simulink model "block_diagram_for_three_phase_csi"  (R2014a)
settings: Solver=ode23t  StartTime=0  StopTime=1  MaxStep=1e-6  RelTol=1e-3
values from neighbouring files (symbols this model uses):
  p11 = rem(m,360)    [code_for_single_phase_csi.m]    (also in code_for_single_phase_vsi.m; code_for_three_phase_csi.m; code_for_three_phase_vsi.m; code_for_vsi.m)
  p22 = rem(n,360)    [code_for_single_phase_csi.m]    (also in code_for_single_phase_vsi.m; code_for_three_phase_csi.m; code_for_three_phase_vsi.m; code_for_vsi.m)
  p33 = rem(o,360)    [code_for_single_phase_csi.m]    (also in code_for_single_phase_vsi.m; code_for_three_phase_csi.m; code_for_three_phase_vsi.m; code_for_vsi.m)
  p44 = rem(p,360)    [code_for_single_phase_csi.m]    (also in code_for_single_phase_vsi.m; code_for_three_phase_csi.m; code_for_three_phase_vsi.m; code_for_vsi.m)
  p55 = rem(q,360)    [code_for_single_phase_csi.m]    (also in code_for_single_phase_vsi.m; code_for_three_phase_csi.m; code_for_three_phase_vsi.m; code_for_vsi.m)
  p66 = rem(r,360)    [code_for_single_phase_csi.m]    (also in code_for_single_phase_vsi.m; code_for_three_phase_csi.m; code_for_three_phase_vsi.m; code_for_vsi.m)
  p77 = rem(s,360)    [code_for_single_phase_csi.m]    (also in code_for_single_phase_vsi.m; code_for_three_phase_csi.m; code_for_three_phase_vsi.m; code_for_vsi.m)
libraries: powerlib x14, powerlib_meascontrol x2
settings Model: Creator=singa  LastModifiedBy=singa

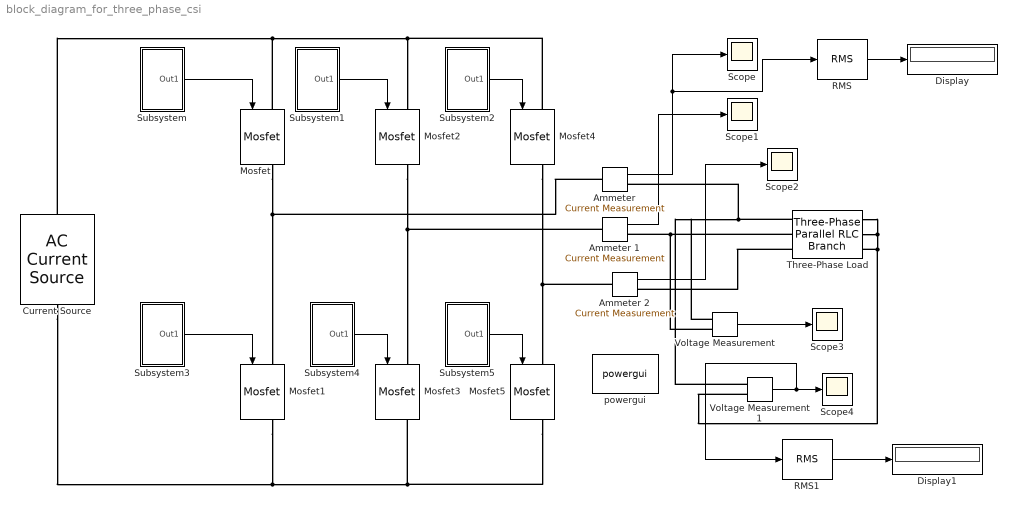
== system block_diagram_for_three_phase_csi ==
  Ammeter : powerlib/Measurements/Current Measurement  PhasorSimulation=off  OutputType=Complex  PSBequivalent=0
  Ammeter 1 : powerlib/Measurements/Current Measurement  PhasorSimulation=off  OutputType=Complex  PSBequivalent=0
  Ammeter 2 : powerlib/Measurements/Current Measurement  PhasorSimulation=off  OutputType=Complex  PSBequivalent=0
  Current Source : powerlib/Electrical Sources/AC Current Source  Amplitude=200  Phase=90  Frequency=0  SampleTime=0  Measurements=None
  Display : Display
  Display1 : Display
  Mosfet{,1..5} (6 alike) : powerlib/Power Electronics/Mosfet  Ron=0.1  Lon=0  Rd=0.01  Vfd=0  IC=0  Rs=1e5  Cs=inf  Measurements=on
  RMS : powerlib_meascontrol/Measurements/RMS  TrueRMS=on  Freq=50  RMSInit=120  Ts=0
  RMS1 : powerlib_meascontrol/Measurements/RMS  TrueRMS=on  Freq=50  RMSInit=120  Ts=0
  Scope{,1..4} (5 alike) : Scope
      Scope settings: YMin=-8  YMax=8  SampleInput=on  SampleTime=1e-6
      Scope1 settings: YMin=-8  YMax=8  SampleInput=on  SampleTime=1e-6
      Scope2 settings: YMin=-8  YMax=8  SaveName=ScopeData2  SampleInput=on  SampleTime=1e-6
      Scope3 settings: YMin=-8  YMax=8  SaveName=ScopeData3  SampleInput=on  SampleTime=1e-6
      Scope4 settings: YMin=-8  YMax=8  SaveName=ScopeData4  SampleInput=on  SampleTime=1e-6
  Subsystem : Subsystem
  Subsystem1 : Subsystem
  Subsystem2 : Subsystem
  Subsystem3 : Subsystem
  Subsystem4 : Subsystem
  Subsystem5 : Subsystem
  Three-Phase Load : powerlib/Elements/Three-Phase Parallel RLC Branch  LConnTagsString=A|B|C  RConnTagsString=A|B|C  BranchType=RC  Resistance=1  Inductance=1e-3  Capacitance=0.1  Measurements=None
  Voltage Measurement : powerlib/Measurements/Voltage Measurement  PhasorSimulation=off  OutputType=Complex  PSBequivalent=0
  Voltage Measurement1 : powerlib/Measurements/Voltage Measurement  PhasorSimulation=off  OutputType=Complex  PSBequivalent=0
  powergui : powerlib/powergui  Priority=1  SimulationMode=Continuous  SolverType=Tustin  SampleTime=50e-6  frequency=60  SPID=off  DisableSnubberDevices=off  DisableRonSwitches=off  DisableVfSwitches=off  SwTol=0  Interpol=off  DisplayEquations=off  Ts=0  methode=off  frequencyindice=0  Pbase=100e6  ErrMax=1e-4  Iterations=50  UnitsV=kV  UnitsW=MW  FunctionMessages=off  echomessages=off  HookPort=off  EnableUseOfTLC=off  x0status=blocks  RestoreLinks=warning  ResistiveCurrentMeasurement=off  Frange=[0:2:500]  Ylog=off  Xlog=on  ShowGrid=off  save=off  variable=ZData  structure=ScopeData  ZoomFFT=off  StartTime=0.8  cycles=2  DisplayStyle=4  fundamental=50  FreqAxis=on  MaxFrequency=2500  frequencyindicesteady=1  RmsSteady=1  display=off
  wires:
  Ammeter/1 -> Scope/1, RMS/1
  Ammeter 1/1 -> Scope1/1
  Ammeter 2/1 -> Scope2/1
  Subsystem/1(Out1) -> Mosfet/1
  Subsystem1/1(Out1) -> Mosfet2/1
  Subsystem2/1(Out1) -> Mosfet4/1
  Subsystem3/1(Out1) -> Mosfet1/1
  Subsystem4/1(Out1) -> Mosfet3/1
  Subsystem5/1(Out1) -> Mosfet5/1
  Voltage Measurement/1 -> Scope3/1
  Voltage Measurement1/1 -> RMS1/1, Scope4/1
  RMS1/1 -> Display1/1
  RMS/1 -> Display/1
  connections:
  Mosfet/RConn1 -- Mosfet1/LConn1 -- Ammeter/LConn1
  Mosfet2/RConn1 -- Mosfet3/LConn1 -- Ammeter 1/LConn1
  Mosfet4/RConn1 -- Ammeter 2/LConn1 -- Mosfet5/LConn1
  Mosfet/LConn1 -- Mosfet4/LConn1 -- Mosfet2/LConn1 -- Current Source/RConn1
  Mosfet1/RConn1 -- Mosfet5/RConn1 -- Mosfet3/RConn1 -- Current Source/LConn1
  Three-Phase Load/LConn1 -- Voltage Measurement1/LConn1 -- Voltage Measurement/LConn1 -- Ammeter/RConn1
  Three-Phase Load/LConn2 -- Voltage Measurement/LConn2 -- Ammeter 1/RConn1
  Three-Phase Load/LConn3 -- Ammeter 2/RConn1
  Three-Phase Load/RConn1 -- Three-Phase Load/RConn2 -- Voltage Measurement1/LConn2 -- Three-Phase Load/RConn3

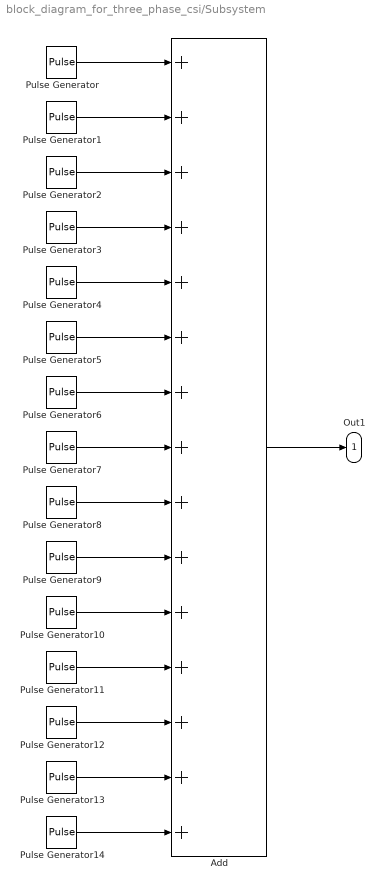
== system block_diagram_for_three_phase_csi/Subsystem ==
  Add : Sum  Inputs=+++++++++++++++
  Pulse Generator : DiscretePulseGenerator  PulseType=Time based  Period=0.02  PulseWidth=(p22-p11)/360*100  PhaseDelay=p11/360*0.02
  Pulse Generator1 : DiscretePulseGenerator  PulseType=Time based  Period=0.02  PulseWidth=(p55-p44)/360*100  PhaseDelay=p44/360*0.02
  Pulse Generator10 : DiscretePulseGenerator  PulseType=Time based  Period=0.02  PulseWidth=(p22-p11)/360*100  PhaseDelay=(180-p22)/360*0.02
  Pulse Generator11 : DiscretePulseGenerator  PulseType=Time based  Period=0.02  PulseWidth=(p33-p22)/360*100  PhaseDelay=(240+p22)/360*0.02
  Pulse Generator12 : DiscretePulseGenerator  PulseType=Time based  Period=0.02  PulseWidth=(p66-p55)/360*100  PhaseDelay=(240+p55)/360*0.02
  Pulse Generator13 : DiscretePulseGenerator  PulseType=Time based  Period=0.02  PulseWidth=(p66-p55)/360*100  PhaseDelay=(300-p66)/360*0.02
  Pulse Generator14 : DiscretePulseGenerator  PulseType=Time based  Period=0.02  PulseWidth=(p33-p22)/360*100  PhaseDelay=(300-p33)/360*0.02
  Pulse Generator2 : DiscretePulseGenerator  PulseType=Time based  Period=0.02  PulseWidth=(30-p77)/360*100  PhaseDelay=p77/360*0.02
  Pulse Generator3 : DiscretePulseGenerator  PulseType=Time based  Period=0.02  PulseWidth=(p77-p66)/360*100  PhaseDelay=(60-p77)/360*0.02
  Pulse Generator4 : DiscretePulseGenerator  PulseType=Time based  Period=0.02  PulseWidth=(p44-p33)/360*100  PhaseDelay=(60-p44)/360*0.02
  Pulse Generator5 : DiscretePulseGenerator  PulseType=Time based  Period=0.02  PulseWidth=(30+p11)/180*100  PhaseDelay=(60-p11)/360*0.02
  Pulse Generator6 : DiscretePulseGenerator  PulseType=Time based  Period=0.02  PulseWidth=(p44-p33)/360*100  PhaseDelay=(120+p33)/360*0.02
  Pulse Generator7 : DiscretePulseGenerator  PulseType=Time based  Period=0.02  PulseWidth=(p77-p66)/360*100  PhaseDelay=(120+p66)/360*0.02
  Pulse Generator8 : DiscretePulseGenerator  PulseType=Time based  Period=0.02  PulseWidth=(30-p77)/360*100  PhaseDelay=150/360*0.02
  Pulse Generator9 : DiscretePulseGenerator  PulseType=Time based  Period=0.02  PulseWidth=(p55-p44)/360*100  PhaseDelay=(180-p55)/360*0.02
  Out1 : Outport
  wires:
  Add/1 -> Out1/1
  Pulse Generator2/1 -> Add/3
  Pulse Generator/1 -> Add/1
  Pulse Generator1/1 -> Add/2
  Pulse Generator3/1 -> Add/4
  Pulse Generator9/1 -> Add/10
  Pulse Generator13/1 -> Add/14
  Pulse Generator14/1 -> Add/15
  Pulse Generator12/1 -> Add/13
  Pulse Generator6/1 -> Add/7
  Pulse Generator7/1 -> Add/8
  Pulse Generator4/1 -> Add/5
  Pulse Generator8/1 -> Add/9
  Pulse Generator11/1 -> Add/12
  Pulse Generator5/1 -> Add/6
  Pulse Generator10/1 -> Add/11

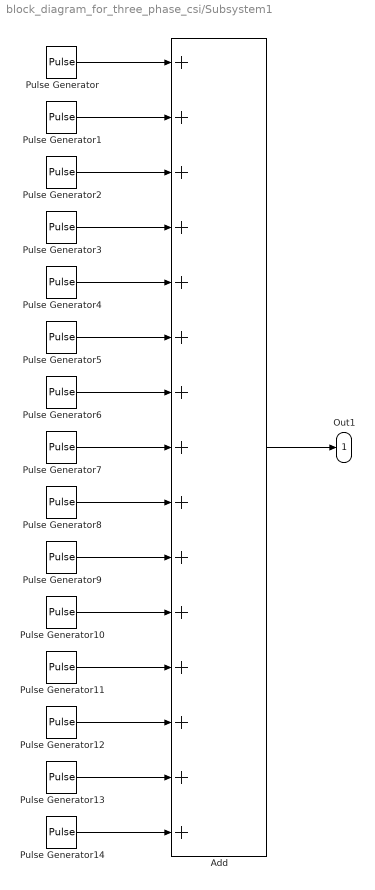
== system block_diagram_for_three_phase_csi/Subsystem1 ==
  Add : Sum  Inputs=+++++++++++++++
  Pulse Generator : DiscretePulseGenerator  PulseType=Time based  Period=0.02  PulseWidth=(p22-p11)/360*100  PhaseDelay=p11/360*0.02+0.02/3
  Pulse Generator1 : DiscretePulseGenerator  PulseType=Time based  Period=0.02  PulseWidth=(p55-p44)/360*100  PhaseDelay=p44/360*0.02+0.02/3
  Pulse Generator10 : DiscretePulseGenerator  PulseType=Time based  Period=0.02  PulseWidth=(p22-p11)/360*100  PhaseDelay=(180-p22)/360*0.02+0.02/3
  Pulse Generator11 : DiscretePulseGenerator  PulseType=Time based  Period=0.02  PulseWidth=(p33-p22)/360*100  PhaseDelay=(240+p22)/360*0.02+0.02/3
  Pulse Generator12 : DiscretePulseGenerator  PulseType=Time based  Period=0.02  PulseWidth=(p66-p55)/360*100  PhaseDelay=(240+p55)/360*0.02+0.02/3
  Pulse Generator13 : DiscretePulseGenerator  PulseType=Time based  Period=0.02  PulseWidth=(p66-p55)/360*100  PhaseDelay=(300-p66)/360*0.02+0.02/3
  Pulse Generator14 : DiscretePulseGenerator  PulseType=Time based  Period=0.02  PulseWidth=(p33-p22)/360*100  PhaseDelay=(300-p33)/360*0.02+0.02/3
  Pulse Generator2 : DiscretePulseGenerator  PulseType=Time based  Period=0.02  PulseWidth=(30-p77)/360*100  PhaseDelay=p77/360*0.02+0.02/3
  Pulse Generator3 : DiscretePulseGenerator  PulseType=Time based  Period=0.02  PulseWidth=(p77-p66)/360*100  PhaseDelay=(60-p77)/360*0.02+0.02/3
  Pulse Generator4 : DiscretePulseGenerator  PulseType=Time based  Period=0.02  PulseWidth=(p44-p33)/360*100  PhaseDelay=(60-p44)/360*0.02+0.02/3
  Pulse Generator5 : DiscretePulseGenerator  PulseType=Time based  Period=0.02  PulseWidth=(30+p11)/180*100  PhaseDelay=(60-p11)/360*0.02+0.02/3
  Pulse Generator6 : DiscretePulseGenerator  PulseType=Time based  Period=0.02  PulseWidth=(p44-p33)/360*100  PhaseDelay=(120+p33)/360*0.02+0.02/3
  Pulse Generator7 : DiscretePulseGenerator  PulseType=Time based  Period=0.02  PulseWidth=(p77-p66)/360*100  PhaseDelay=(120+p66)/360*0.02+0.02/3
  Pulse Generator8 : DiscretePulseGenerator  PulseType=Time based  Period=0.02  PulseWidth=(30-p77)/360*100  PhaseDelay=150/360*0.02+0.02/3
  Pulse Generator9 : DiscretePulseGenerator  PulseType=Time based  Period=0.02  PulseWidth=(p55-p44)/360*100  PhaseDelay=(180-p55)/360*0.02+0.02/3
  Out1 : Outport
  wires:
  Pulse Generator2/1 -> Add/3
  Pulse Generator/1 -> Add/1
  Pulse Generator1/1 -> Add/2
  Pulse Generator3/1 -> Add/4
  Pulse Generator9/1 -> Add/10
  Pulse Generator13/1 -> Add/14
  Pulse Generator14/1 -> Add/15
  Pulse Generator12/1 -> Add/13
  Pulse Generator6/1 -> Add/7
  Pulse Generator7/1 -> Add/8
  Pulse Generator4/1 -> Add/5
  Pulse Generator8/1 -> Add/9
  Pulse Generator11/1 -> Add/12
  Pulse Generator5/1 -> Add/6
  Pulse Generator10/1 -> Add/11
  Add/1 -> Out1/1

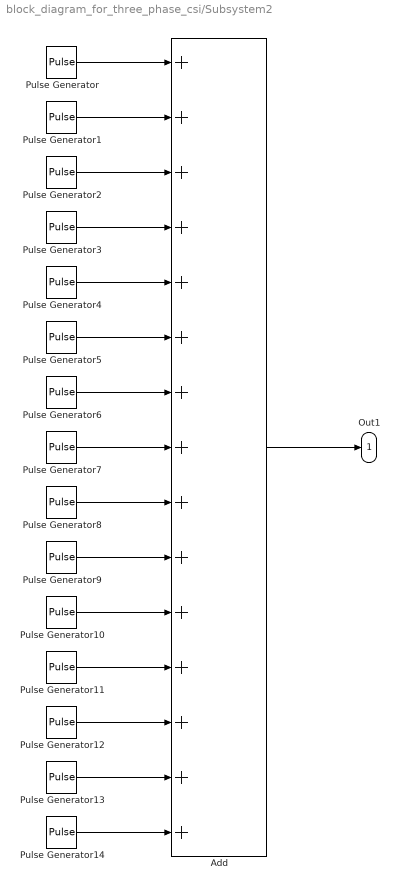
== system block_diagram_for_three_phase_csi/Subsystem2 ==
  Add : Sum  Inputs=+++++++++++++++
  Pulse Generator : DiscretePulseGenerator  PulseType=Time based  Period=0.02  PulseWidth=(p22-p11)/360*100  PhaseDelay=p11/360*0.02+0.04/3
  Pulse Generator1 : DiscretePulseGenerator  PulseType=Time based  Period=0.02  PulseWidth=(p55-p44)/360*100  PhaseDelay=p44/360*0.02+0.04/3
  Pulse Generator10 : DiscretePulseGenerator  PulseType=Time based  Period=0.02  PulseWidth=(p22-p11)/360*100  PhaseDelay=(180-p22)/360*0.02+0.04/3
  Pulse Generator11 : DiscretePulseGenerator  PulseType=Time based  Period=0.02  PulseWidth=(p33-p22)/360*100  PhaseDelay=(240+p22)/360*0.02+0.04/3
  Pulse Generator12 : DiscretePulseGenerator  PulseType=Time based  Period=0.02  PulseWidth=(p66-p55)/360*100  PhaseDelay=(240+p55)/360*0.02+0.04/3
  Pulse Generator13 : DiscretePulseGenerator  PulseType=Time based  Period=0.02  PulseWidth=(p66-p55)/360*100  PhaseDelay=(300-p66)/360*0.02+0.04/3
  Pulse Generator14 : DiscretePulseGenerator  PulseType=Time based  Period=0.02  PulseWidth=(p33-p22)/360*100  PhaseDelay=(300-p33)/360*0.02+0.04/3
  Pulse Generator2 : DiscretePulseGenerator  PulseType=Time based  Period=0.02  PulseWidth=(30-p77)/360*100  PhaseDelay=p77/360*0.02+0.04/3
  Pulse Generator3 : DiscretePulseGenerator  PulseType=Time based  Period=0.02  PulseWidth=(p77-p66)/360*100  PhaseDelay=(60-p77)/360*0.02+0.04/3
  Pulse Generator4 : DiscretePulseGenerator  PulseType=Time based  Period=0.02  PulseWidth=(p44-p33)/360*100  PhaseDelay=(60-p44)/360*0.02+0.04/3
  Pulse Generator5 : DiscretePulseGenerator  PulseType=Time based  Period=0.02  PulseWidth=(30+p11)/180*100  PhaseDelay=(60-p11)/360*0.02+0.04/3
  Pulse Generator6 : DiscretePulseGenerator  PulseType=Time based  Period=0.02  PulseWidth=(p44-p33)/360*100  PhaseDelay=(120+p33)/360*0.02+0.04/3
  Pulse Generator7 : DiscretePulseGenerator  PulseType=Time based  Period=0.02  PulseWidth=(p77-p66)/360*100  PhaseDelay=(120+p66)/360*0.02+0.04/3
  Pulse Generator8 : DiscretePulseGenerator  PulseType=Time based  Period=0.02  PulseWidth=(30-p77)/360*100  PhaseDelay=150/360*0.02+0.04/3
  Pulse Generator9 : DiscretePulseGenerator  PulseType=Time based  Period=0.02  PulseWidth=(p55-p44)/360*100  PhaseDelay=(180-p55)/360*0.02+0.04/3
  Out1 : Outport
  wires:
  Pulse Generator2/1 -> Add/3
  Pulse Generator/1 -> Add/1
  Pulse Generator1/1 -> Add/2
  Pulse Generator3/1 -> Add/4
  Pulse Generator9/1 -> Add/10
  Pulse Generator13/1 -> Add/14
  Pulse Generator14/1 -> Add/15
  Pulse Generator12/1 -> Add/13
  Pulse Generator6/1 -> Add/7
  Pulse Generator7/1 -> Add/8
  Pulse Generator4/1 -> Add/5
  Pulse Generator8/1 -> Add/9
  Pulse Generator11/1 -> Add/12
  Pulse Generator5/1 -> Add/6
  Pulse Generator10/1 -> Add/11
  Add/1 -> Out1/1

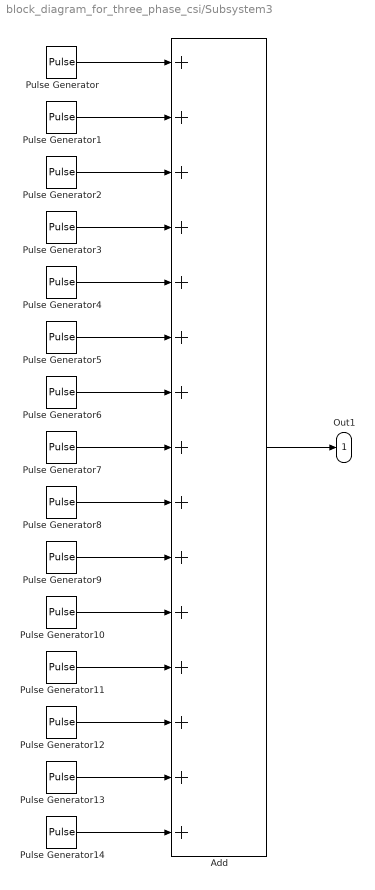
== system block_diagram_for_three_phase_csi/Subsystem3 ==
  Add : Sum  Inputs=+++++++++++++++
  Pulse Generator : DiscretePulseGenerator  PulseType=Time based  Period=0.02  PulseWidth=(p22-p11)/360*100  PhaseDelay=p11/360*0.02+0.01
  Pulse Generator1 : DiscretePulseGenerator  PulseType=Time based  Period=0.02  PulseWidth=(p55-p44)/360*100  PhaseDelay=p44/360*0.02+0.01
  Pulse Generator10 : DiscretePulseGenerator  PulseType=Time based  Period=0.02  PulseWidth=(p22-p11)/360*100  PhaseDelay=(180-p22)/360*0.02+0.01
  Pulse Generator11 : DiscretePulseGenerator  PulseType=Time based  Period=0.02  PulseWidth=(p33-p22)/360*100  PhaseDelay=(240+p22)/360*0.02+0.01
  Pulse Generator12 : DiscretePulseGenerator  PulseType=Time based  Period=0.02  PulseWidth=(p66-p55)/360*100  PhaseDelay=(240+p55)/360*0.02+0.01
  Pulse Generator13 : DiscretePulseGenerator  PulseType=Time based  Period=0.02  PulseWidth=(p66-p55)/360*100  PhaseDelay=(300-p66)/360*0.02+0.01
  Pulse Generator14 : DiscretePulseGenerator  PulseType=Time based  Period=0.02  PulseWidth=(p33-p22)/360*100  PhaseDelay=(300-p33)/360*0.02+0.01
  Pulse Generator2 : DiscretePulseGenerator  PulseType=Time based  Period=0.02  PulseWidth=(30-p77)/360*100  PhaseDelay=p77/360*0.02+0.01
  Pulse Generator3 : DiscretePulseGenerator  PulseType=Time based  Period=0.02  PulseWidth=(p77-p66)/360*100  PhaseDelay=(60-p77)/360*0.02+0.01
  Pulse Generator4 : DiscretePulseGenerator  PulseType=Time based  Period=0.02  PulseWidth=(p44-p33)/360*100  PhaseDelay=(60-p44)/360*0.02+0.01
  Pulse Generator5 : DiscretePulseGenerator  PulseType=Time based  Period=0.02  PulseWidth=(30+p11)/180*100  PhaseDelay=(60-p11)/360*0.02+0.01
  Pulse Generator6 : DiscretePulseGenerator  PulseType=Time based  Period=0.02  PulseWidth=(p44-p33)/360*100  PhaseDelay=(120+p33)/360*0.02+0.01
  Pulse Generator7 : DiscretePulseGenerator  PulseType=Time based  Period=0.02  PulseWidth=(p77-p66)/360*100  PhaseDelay=(120+p66)/360*0.02+0.01
  Pulse Generator8 : DiscretePulseGenerator  PulseType=Time based  Period=0.02  PulseWidth=(30-p77)/360*100  PhaseDelay=150/360*0.02+0.01
  Pulse Generator9 : DiscretePulseGenerator  PulseType=Time based  Period=0.02  PulseWidth=(p55-p44)/360*100  PhaseDelay=(180-p55)/360*0.02+0.01
  Out1 : Outport
  wires:
  Pulse Generator2/1 -> Add/3
  Pulse Generator/1 -> Add/1
  Pulse Generator1/1 -> Add/2
  Pulse Generator3/1 -> Add/4
  Pulse Generator9/1 -> Add/10
  Pulse Generator13/1 -> Add/14
  Pulse Generator14/1 -> Add/15
  Pulse Generator12/1 -> Add/13
  Pulse Generator6/1 -> Add/7
  Pulse Generator7/1 -> Add/8
  Pulse Generator4/1 -> Add/5
  Pulse Generator8/1 -> Add/9
  Pulse Generator11/1 -> Add/12
  Pulse Generator5/1 -> Add/6
  Pulse Generator10/1 -> Add/11
  Add/1 -> Out1/1

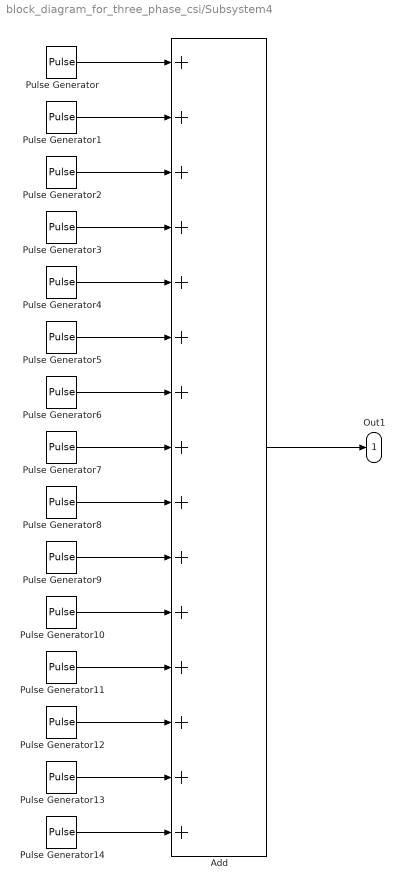
== system block_diagram_for_three_phase_csi/Subsystem4 ==
  Add : Sum  Inputs=+++++++++++++++
  Pulse Generator : DiscretePulseGenerator  PulseType=Time based  Period=0.02  PulseWidth=(p22-p11)/360*100  PhaseDelay=p11/360*0.02+0.01+0.02/3
  Pulse Generator1 : DiscretePulseGenerator  PulseType=Time based  Period=0.02  PulseWidth=(p55-p44)/360*100  PhaseDelay=p44/360*0.02+0.01+0.02/3
  Pulse Generator10 : DiscretePulseGenerator  PulseType=Time based  Period=0.02  PulseWidth=(p22-p11)/360*100  PhaseDelay=(180-p22)/360*0.02+0.01+0.02/3
  Pulse Generator11 : DiscretePulseGenerator  PulseType=Time based  Period=0.02  PulseWidth=(p33-p22)/360*100  PhaseDelay=(240+p22)/360*0.02+0.01+0.02/3
  Pulse Generator12 : DiscretePulseGenerator  PulseType=Time based  Period=0.02  PulseWidth=(p66-p55)/360*100  PhaseDelay=(240+p55)/360*0.02+0.01+0.02/3
  Pulse Generator13 : DiscretePulseGenerator  PulseType=Time based  Period=0.02  PulseWidth=(p66-p55)/360*100  PhaseDelay=(300-p66)/360*0.02+0.01+0.02/3
  Pulse Generator14 : DiscretePulseGenerator  PulseType=Time based  Period=0.02  PulseWidth=(p33-p22)/360*100  PhaseDelay=(300-p33)/360*0.02+0.01+0.02/3
  Pulse Generator2 : DiscretePulseGenerator  PulseType=Time based  Period=0.02  PulseWidth=(30-p77)/360*100  PhaseDelay=p77/360*0.02+0.01+0.02/3
  Pulse Generator3 : DiscretePulseGenerator  PulseType=Time based  Period=0.02  PulseWidth=(p77-p66)/360*100  PhaseDelay=(60-p77)/360*0.02+0.01+0.02/3
  Pulse Generator4 : DiscretePulseGenerator  PulseType=Time based  Period=0.02  PulseWidth=(p44-p33)/360*100  PhaseDelay=(60-p44)/360*0.02+0.01+0.02/3
  Pulse Generator5 : DiscretePulseGenerator  PulseType=Time based  Period=0.02  PulseWidth=(30+p11)/180*100  PhaseDelay=(60-p11)/360*0.02+0.01+0.02/3
  Pulse Generator6 : DiscretePulseGenerator  PulseType=Time based  Period=0.02  PulseWidth=(p44-p33)/360*100  PhaseDelay=(120+p33)/360*0.02+0.01+0.02/3
  Pulse Generator7 : DiscretePulseGenerator  PulseType=Time based  Period=0.02  PulseWidth=(p77-p66)/360*100  PhaseDelay=(120+p66)/360*0.02+0.01+0.02/3
  Pulse Generator8 : DiscretePulseGenerator  PulseType=Time based  Period=0.02  PulseWidth=(30-p77)/360*100  PhaseDelay=150/360*0.02+0.01+0.02/3
  Pulse Generator9 : DiscretePulseGenerator  PulseType=Time based  Period=0.02  PulseWidth=(p55-p44)/360*100  PhaseDelay=(180-p55)/360*0.02+0.01+0.02/3
  Out1 : Outport
  wires:
  Pulse Generator2/1 -> Add/3
  Pulse Generator/1 -> Add/1
  Pulse Generator1/1 -> Add/2
  Pulse Generator3/1 -> Add/4
  Pulse Generator9/1 -> Add/10
  Pulse Generator13/1 -> Add/14
  Pulse Generator14/1 -> Add/15
  Pulse Generator12/1 -> Add/13
  Pulse Generator6/1 -> Add/7
  Pulse Generator7/1 -> Add/8
  Pulse Generator4/1 -> Add/5
  Pulse Generator8/1 -> Add/9
  Pulse Generator11/1 -> Add/12
  Pulse Generator5/1 -> Add/6
  Pulse Generator10/1 -> Add/11
  Add/1 -> Out1/1

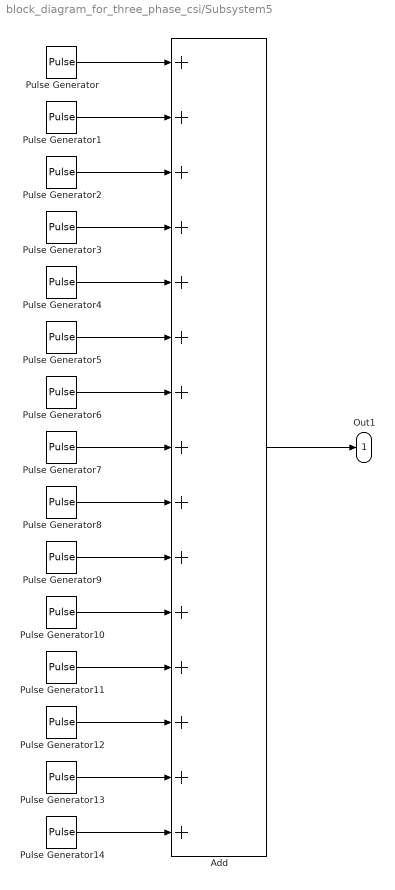
== system block_diagram_for_three_phase_csi/Subsystem5 ==
  Add : Sum  Inputs=+++++++++++++++
  Pulse Generator : DiscretePulseGenerator  PulseType=Time based  Period=0.02  PulseWidth=(p22-p11)/360*100  PhaseDelay=p11/360*0.02+0.01+0.04/3
  Pulse Generator1 : DiscretePulseGenerator  PulseType=Time based  Period=0.02  PulseWidth=(p55-p44)/360*100  PhaseDelay=p44/360*0.02+0.01+0.04/3
  Pulse Generator10 : DiscretePulseGenerator  PulseType=Time based  Period=0.02  PulseWidth=(p22-p11)/360*100  PhaseDelay=(180-p22)/360*0.02+0.01+0.04/3
  Pulse Generator11 : DiscretePulseGenerator  PulseType=Time based  Period=0.02  PulseWidth=(p33-p22)/360*100  PhaseDelay=(240+p22)/360*0.02+0.01+0.04/3
  Pulse Generator12 : DiscretePulseGenerator  PulseType=Time based  Period=0.02  PulseWidth=(p66-p55)/360*100  PhaseDelay=(240+p55)/360*0.02+0.01+0.04/3
  Pulse Generator13 : DiscretePulseGenerator  PulseType=Time based  Period=0.02  PulseWidth=(p66-p55)/360*100  PhaseDelay=(300-p66)/360*0.02+0.01+0.04/3
  Pulse Generator14 : DiscretePulseGenerator  PulseType=Time based  Period=0.02  PulseWidth=(p33-p22)/360*100  PhaseDelay=(300-p33)/360*0.02+0.01+0.04/3
  Pulse Generator2 : DiscretePulseGenerator  PulseType=Time based  Period=0.02  PulseWidth=(30-p77)/360*100  PhaseDelay=p77/360*0.02+0.01+0.04/3
  Pulse Generator3 : DiscretePulseGenerator  PulseType=Time based  Period=0.02  PulseWidth=(p77-p66)/360*100  PhaseDelay=(60-p77)/360*0.02+0.01+0.04/3
  Pulse Generator4 : DiscretePulseGenerator  PulseType=Time based  Period=0.02  PulseWidth=(p44-p33)/360*100  PhaseDelay=(60-p44)/360*0.02+0.01+0.04/3
  Pulse Generator5 : DiscretePulseGenerator  PulseType=Time based  Period=0.02  PulseWidth=(30+p11)/180*100  PhaseDelay=(60-p11)/360*0.02+0.01+0.04/3
  Pulse Generator6 : DiscretePulseGenerator  PulseType=Time based  Period=0.02  PulseWidth=(p44-p33)/360*100  PhaseDelay=(120+p33)/360*0.02+0.01+0.04/3
  Pulse Generator7 : DiscretePulseGenerator  PulseType=Time based  Period=0.02  PulseWidth=(p77-p66)/360*100  PhaseDelay=(120+p66)/360*0.02+0.01+0.04/3
  Pulse Generator8 : DiscretePulseGenerator  PulseType=Time based  Period=0.02  PulseWidth=(30-p77)/360*100  PhaseDelay=150/360*0.02+0.01+0.04/3
  Pulse Generator9 : DiscretePulseGenerator  PulseType=Time based  Period=0.02  PulseWidth=(p55-p44)/360*100  PhaseDelay=(180-p55)/360*0.02+0.01+0.04/3
  Out1 : Outport
  wires:
  Pulse Generator2/1 -> Add/3
  Pulse Generator/1 -> Add/1
  Pulse Generator1/1 -> Add/2
  Pulse Generator3/1 -> Add/4
  Pulse Generator9/1 -> Add/10
  Pulse Generator13/1 -> Add/14
  Pulse Generator14/1 -> Add/15
  Pulse Generator12/1 -> Add/13
  Pulse Generator6/1 -> Add/7
  Pulse Generator7/1 -> Add/8
  Pulse Generator4/1 -> Add/5
  Pulse Generator8/1 -> Add/9
  Pulse Generator11/1 -> Add/12
  Pulse Generator5/1 -> Add/6
  Pulse Generator10/1 -> Add/11
  Add/1 -> Out1/1
